simulink library "makeBcW_cl"  (R2020a)
settings: Solver=VariableStepAuto  StartTime=0.0  StopTime=10.0  RelTol=1e-3
libraries: rotationAboutY x1, rotationAboutZ x1
settings Model: Creator=Ayaz  LastModifiedBy=Ayaz

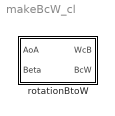
== system makeBcW_cl ==
  rotationBtoW : Subsystem

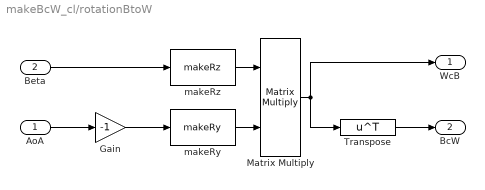
== system makeBcW_cl/rotationBtoW ==
  AoA : Inport
  Beta : Inport  Port=2
  Gain : Gain  Gain=-1
  Matrix Multiply : Product  Multiplication=Matrix(*)
  Transpose : Math  Operator=transpose  SaturateOnIntegerOverflow=on
  makeRy : rotationAboutY/makeRy  SystemSampleTime=-1  Latency=0  AutoFrameSizeCalculation=off
  makeRz : rotationAboutZ/makeRz  SystemSampleTime=-1  Latency=0  AutoFrameSizeCalculation=off
  WcB : Outport
  BcW : Outport  Port=2
  wires:
  Matrix Multiply/1 -> WcB/1, Transpose/1
  Transpose/1 -> BcW/1
  AoA/1 -> Gain/1
  Gain/1 -> makeRy/1
  Beta/1 -> makeRz/1
  makeRz/1 -> Matrix Multiply/1
  makeRy/1 -> Matrix Multiply/2
